simulink model "SecRwLtStArmScrnCtrl"  (R2018b)
settings: Solver=FixedStepDiscrete  StartTime=0.0  StopTime=10.0  FixedStep=0.01  RelTol=1e-3
undefined symbols (not defined in the file or in its folder): KeSMSuMdMotFinshdTm_Val, KeSMSuMdRetryTm1_Val, KeSMSuModeReqDurgTm_Val, KeSMSwSecRwLtStArmScrnEnTrigBitMask_Val
libraries: StCtrlLib x1
settings Model: Creator=sn2xws  LastModifiedBy=sn2xws
settings DataIOCC: SaveFormat=StructureWithTime
settings OptimizationCC: DefaultParameterBehavior=Inlined  EnhancedBackFolding=on  PassReuseOutputArgsAs=Individual arguments  ZeroExternalMemoryAtStartup=off  ZeroInternalMemoryAtStartup=off  OptimizeBlockOrder=speed  DifferentSizesBufferReuse=on  OptimizationCustomize=off
settings DebuggingCC: ParameterTunabilityLossMsg=error
settings ModelReferenceCC: ModelReferenceNumInstancesAllowed=Single
settings SFSimCC: MATLABDynamicMemAlloc=off
settings RTWCC: SystemTargetFile=autosar.tlc  GenCodeOnly=on  TemplateMakefile=ert_default_tmf  Description=AUTOSAR  GenerateReport=on  IncludeHyperlinkInReport=on  LaunchReport=on  GenerateTraceInfo=on  GenerateTraceReport=on  GenerateTraceReportSl=on  GenerateTraceReportSf=on  GenerateTraceReportEml=on
settings CodeAppCC: ForceParamTrailComments=on  IgnoreCustomStorageClasses=off  OperatorAnnotations=on  SimulinkDataObjDesc=on  SFDataObjDesc=on  InsertBlockDesc=on
settings STFCustomTargetCC: TargetLangStandard=C99 (ISO)  MultiwordLength=256  ParMdlRefBuildCompliant=on  CompOptLevelCompliant=on  IncludeMdlTerminateFcn=off  CombineOutputUpdateFcns=on  SuppressErrorStatus=on  ERTCustomFileBanners=on  SupportNonFinite=off  SupportComplex=off  SupportContinuousTime=off  SupportNonInlinedSFcns=off  RemoveResetFunc=on  MATLABClassNameForMDSCustomization=Simulink.SoftwareTarget.ERTCustomization  AutosarCompliant=on  UseToolchainInfoCompliant=on  LookupTableObjectStructAxisOrder=2,1,3,4,...  LUTObjectStructOrderEvenSpacing=Size,Table,Breakpoints  SystemTargetFile=autosar.tlc
settings ERTTargetCC: TargetLangStandard=C99 (ISO)  ConcurrentExecutionCompliant=off  IncludeMdlTerminateFcn=off  SuppressErrorStatus=on  SupportNonFinite=off  SupportComplex=off  ModelStepFunctionPrototypeControlCompliant=off  CPPClassGenCompliant=off  AutosarCompliant=on  LookupTableObjectStructAxisOrder=2,1,3,4,...  LUTObjectStructOrderEvenSpacing=Size,Table,Breakpoints  InlinedParameterPlacement=NonHierarchical  ERTCustomFileTemplate=example_file_process.tlc  ERTFilePackagingFormat=Compact

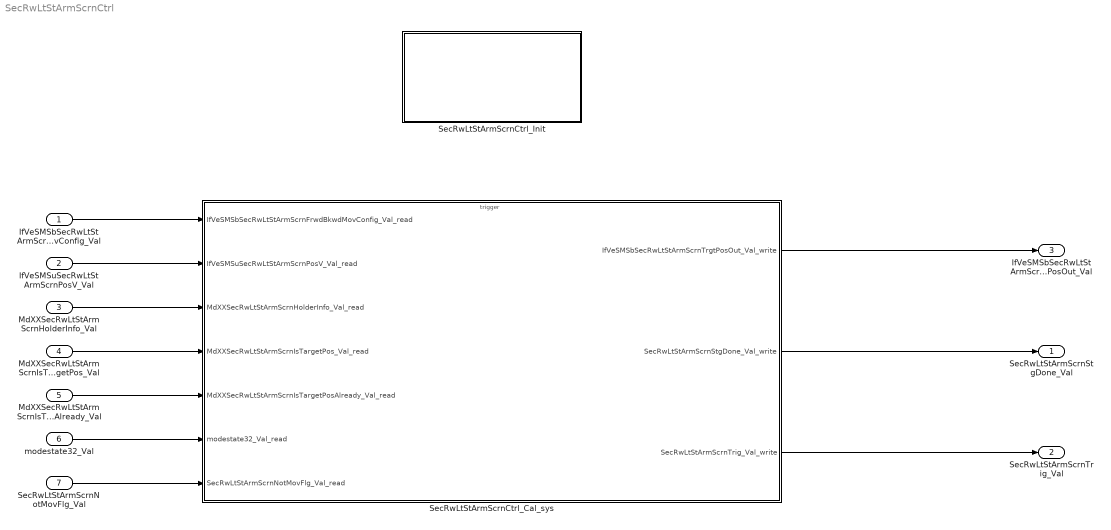
== system SecRwLtStArmScrnCtrl ==
  IfVeSMSbSecRwLtStArmScrnFrwdBkwdMovConfig_Val : Inport  OutDataTypeStr=boolean  PortDimensions=1
  IfVeSMSuSecRwLtStArmScrnPosV_Val : Inport  Port=2  OutDataTypeStr=boolean  PortDimensions=1
  MdXXSecRwLtStArmScrnHolderInfo_Val : Inport  Port=3  OutDataTypeStr=uint32  PortDimensions=1
  MdXXSecRwLtStArmScrnIsTargetPos_Val : Inport  Port=4  OutDataTypeStr=uint32  PortDimensions=1
  MdXXSecRwLtStArmScrnIsTargetPosAlready_Val : Inport  Port=5  OutDataTypeStr=uint32  PortDimensions=1
  modestate32_Val : Inport  Port=6  OutDataTypeStr=uint32  PortDimensions=1
  SecRwLtStArmScrnNotMovFlg_Val : Inport  Port=7  OutDataTypeStr=boolean  PortDimensions=1
  SecRwLtStArmScrnCtrl_Cal_sys : Subsystem
  SecRwLtStArmScrnCtrl_Init : Subsystem
  SecRwLtStArmScrnStgDone_Val : Outport  OutDataTypeStr=boolean  PortDimensions=1
  SecRwLtStArmScrnTrig_Val : Outport  Port=2  OutDataTypeStr=boolean  PortDimensions=1
  IfVeSMSbSecRwLtStArmScrnTrgtPosOut_Val : Outport  Port=3  OutDataTypeStr=boolean  PortDimensions=1
  wires:
  IfVeSMSbSecRwLtStArmScrnFrwdBkwdMovConfig_Val/1 -> SecRwLtStArmScrnCtrl_Cal_sys/1(IfVeSMSbSecRwLtStArmScrnFrwdBkwdMovConfig_Val_read)
  IfVeSMSuSecRwLtStArmScrnPosV_Val/1 -> SecRwLtStArmScrnCtrl_Cal_sys/2(IfVeSMSuSecRwLtStArmScrnPosV_Val_read)
  MdXXSecRwLtStArmScrnHolderInfo_Val/1 -> SecRwLtStArmScrnCtrl_Cal_sys/3(MdXXSecRwLtStArmScrnHolderInfo_Val_read)
  MdXXSecRwLtStArmScrnIsTargetPos_Val/1 -> SecRwLtStArmScrnCtrl_Cal_sys/4(MdXXSecRwLtStArmScrnIsTargetPos_Val_read)
  MdXXSecRwLtStArmScrnIsTargetPosAlready_Val/1 -> SecRwLtStArmScrnCtrl_Cal_sys/5(MdXXSecRwLtStArmScrnIsTargetPosAlready_Val_read)
  modestate32_Val/1 -> SecRwLtStArmScrnCtrl_Cal_sys/6(modestate32_Val_read)
  SecRwLtStArmScrnNotMovFlg_Val/1 -> SecRwLtStArmScrnCtrl_Cal_sys/7(SecRwLtStArmScrnNotMovFlg_Val_read)
  SecRwLtStArmScrnCtrl_Cal_sys/1(IfVeSMSbSecRwLtStArmScrnTrgtPosOut_Val_write) -> IfVeSMSbSecRwLtStArmScrnTrgtPosOut_Val/1
  SecRwLtStArmScrnCtrl_Cal_sys/2(SecRwLtStArmScrnStgDone_Val_write) -> SecRwLtStArmScrnStgDone_Val/1
  SecRwLtStArmScrnCtrl_Cal_sys/3(SecRwLtStArmScrnTrig_Val_write) -> SecRwLtStArmScrnTrig_Val/1

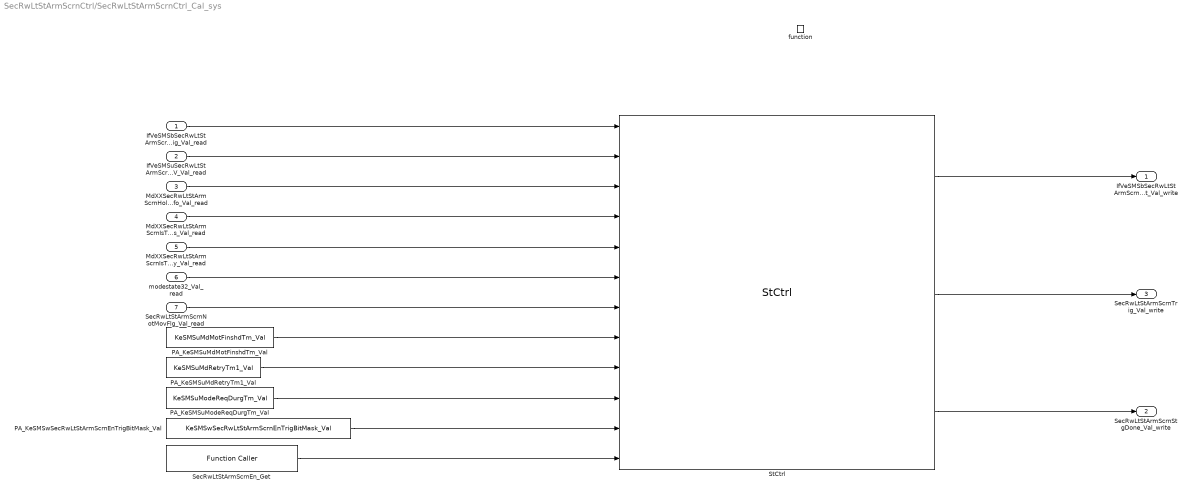
== system SecRwLtStArmScrnCtrl/SecRwLtStArmScrnCtrl_Cal_sys ==
  IfVeSMSbSecRwLtStArmScrnFrwdBkwdMovConfig_Val_read : Inport
  IfVeSMSuSecRwLtStArmScrnPosV_Val_read : Inport  Port=2
  MdXXSecRwLtStArmScrnHolderInfo_Val_read : Inport  Port=3
  MdXXSecRwLtStArmScrnIsTargetPos_Val_read : Inport  Port=4
  MdXXSecRwLtStArmScrnIsTargetPosAlready_Val_read : Inport  Port=5
  modestate32_Val_read : Inport  Port=6
  SecRwLtStArmScrnNotMovFlg_Val_read : Inport  Port=7
  function : TriggerPort  TriggerType=function-call  IsSimulinkFunction=on  FunctionName=SecRwLtStArmScrnCtrl_Cal  VariantControl=(inherit)
  PA_KeSMSuMdMotFinshdTm_Val : Constant  Value=KeSMSuMdMotFinshdTm_Val
  PA_KeSMSuMdRetryTm1_Val : Constant  Value=KeSMSuMdRetryTm1_Val
  PA_KeSMSuModeReqDurgTm_Val : Constant  Value=KeSMSuModeReqDurgTm_Val
  PA_KeSMSwSecRwLtStArmScrnEnTrigBitMask_Val : Constant  Value=KeSMSwSecRwLtStArmScrnEnTrigBitMask_Val
  SecRwLtStArmScrnEn_Get : FunctionCaller  FunctionPrototype=data = SecRwLtStArmScrnEn_Get()  OutputArgumentSpecifications=uint32(1)
  StCtrl : StCtrlLib/StCtrl  SystemSampleTime=-1
  IfVeSMSbSecRwLtStArmScrnTrgtPosOut_Val_write : Outport
      settings: EnsureOutportIsVirtual=on
  SecRwLtStArmScrnStgDone_Val_write : Outport  Port=2
      settings: EnsureOutportIsVirtual=on
  SecRwLtStArmScrnTrig_Val_write : Outport  Port=3
      settings: EnsureOutportIsVirtual=on
  wires:
  StCtrl/1 -> IfVeSMSbSecRwLtStArmScrnTrgtPosOut_Val_write/1
  StCtrl/3 -> SecRwLtStArmScrnStgDone_Val_write/1
  StCtrl/2 -> SecRwLtStArmScrnTrig_Val_write/1
  PA_KeSMSwSecRwLtStArmScrnEnTrigBitMask_Val/1 -> StCtrl/11
  SecRwLtStArmScrnEn_Get/1 -> StCtrl/12
  PA_KeSMSuMdMotFinshdTm_Val/1 -> StCtrl/8
  PA_KeSMSuModeReqDurgTm_Val/1 -> StCtrl/10
  PA_KeSMSuMdRetryTm1_Val/1 -> StCtrl/9
  MdXXSecRwLtStArmScrnHolderInfo_Val_read/1 -> StCtrl/3
  MdXXSecRwLtStArmScrnIsTargetPos_Val_read/1 -> StCtrl/4
  IfVeSMSuSecRwLtStArmScrnPosV_Val_read/1 -> StCtrl/2
  MdXXSecRwLtStArmScrnIsTargetPosAlready_Val_read/1 -> StCtrl/5
  IfVeSMSbSecRwLtStArmScrnFrwdBkwdMovConfig_Val_read/1 -> StCtrl/1
  modestate32_Val_read/1 -> StCtrl/6
  SecRwLtStArmScrnNotMovFlg_Val_read/1 -> StCtrl/7

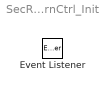
== system SecRwLtStArmScrnCtrl/SecRwLtStArmScrnCtrl_Init ==
  Event Listener : EventListener  EventName=reset
